simulink model "model2MikolajOgarek"  (R2018b)
settings: Solver=ode4  StartTime=0.0  StopTime=10.0  FixedStep=1e-2  RelTol=1e-3
values from neighbouring files (symbols this model uses):
  A = [0,1;-7,-6]    [Mikolaj_Ogarek_Lab3.m]
  Ap = expm(h*A)    [Mikolaj_Ogarek_Lab3.m]
  B = [0;1]    [Mikolaj_Ogarek_Lab3.m]
  Bp = double(int(expm(t*A)*B,t,0,h))    [Mikolaj_Ogarek_Lab3.m]
  C = eye(2)    [Mikolaj_Ogarek_Lab3.m]
  Cp = C    [Mikolaj_Ogarek_Lab3.m]
  h = 0.1    [Mikolaj_Ogarek_Lab3.m]
settings Model: Creator=mikolaj  LastModifiedBy=mikolaj

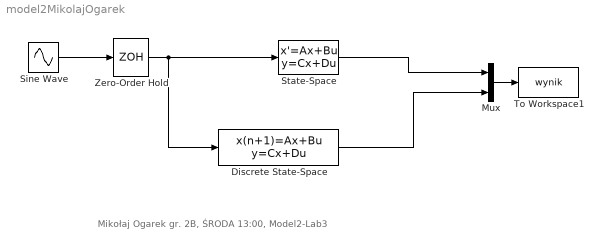
== system model2MikolajOgarek ==
  note: Mikołaj Ogarek gr. 2B, ŚRODA 13:00, Model2-Lab3
  Discrete State-Space : DiscreteStateSpace  A=Ap  B=Bp  C=Cp  D=[0;0]  SampleTime=h
  Mux : Mux  Inputs=2
  Sine Wave : Sin  SampleTime=0
  State-Space : StateSpace  A=A  B=B  C=C  D=[0;0]  InitialCondition=0
  To Workspace1 : ToWorkspace  VariableName=wynik  SampleTime=-1
  Zero-Order Hold : ZeroOrderHold  SampleTime=h
  wires:
  Zero-Order Hold/1 -> State-Space/1, Discrete State-Space/1
  Sine Wave/1 -> Zero-Order Hold/1
  State-Space/1 -> Mux/1
  Mux/1 -> To Workspace1/1
  Discrete State-Space/1 -> Mux/2
